simulink model "Saucer_LQG"  (R2015b)
settings: Solver=ode3  StartTime=0.0  StopTime=inf  FixedStep=0.05  RelTol=1e-3
undefined symbols (not defined in the file or in its folder): A, B, C, K_lqr, Kd, Kp, L_obs, MAPP1, MAPP2, MAPP3, pinvTr, ref, Th1, Th2, Th3
libraries: robotlib x11, realtime_pacer_lib x1
settings Model: Creator=saucer  LastModifiedBy=saucer
settings OptimizationCC: OptimizeModelRefInitCode=on  LifeSpan=Inf  MaxStackSize=64
settings HardwareCC: ProdBitPerPointer=32  ProdLargestAtomicFloat=None  ProdIntDivRoundTo=Undefined  ProdEndianess=Unspecified  ProdWordSize=32  ProdHWDeviceType=Generic->Unspecified (assume 32-bit Generic)
settings RTWCC: SystemTargetFile=ert.tlc  TemplateMakefile=ert_default_tmf  Description=Embedded Coder  Toolchain=Catkin  TargetLang=C++
settings CodeAppCC: IgnoreCustomStorageClasses=off

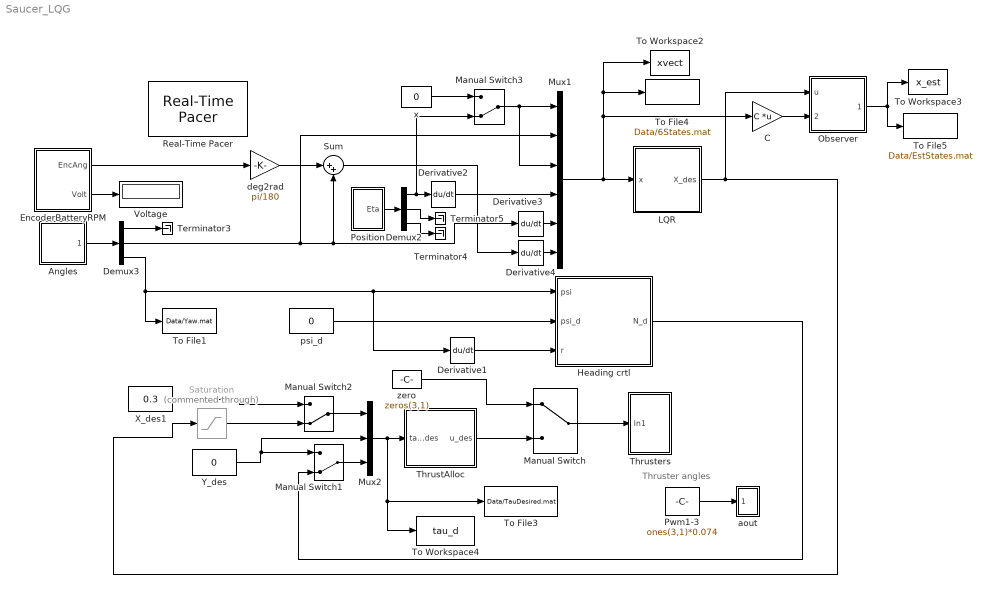
== system Saucer_LQG ==
  note: Thruster angles
  Angles : Subsystem
  C : Gain  Gain=C  Multiplication=Matrix(K*u)
  Demux2 : Demux  Outputs=3
  Demux3 : Demux  Outputs=3
  Derivative{1..4} (4 alike) : Derivative
  EncoderBatteryRPM : Subsystem
  Heading crtl : Subsystem
  LQR : Subsystem
  Manual Switch : ManualSwitch
  Manual Switch1 : ManualSwitch  CurrentSetting=0
  Manual Switch2 : ManualSwitch  CurrentSetting=0
  Manual Switch3 : ManualSwitch  CurrentSetting=0
  Mux1 : Mux  Inputs=6
  Mux2 : Mux  Inputs=3
  Observer : Subsystem
  Position : Subsystem
  Pwm1-3 : Constant  Value=ones(3,1)*0.074
  Real-Time Pacer : realtime_pacer_lib/Real-Time Pacer  simTimePerRealTime=1
  Saturation : Saturate  Commented=through  UpperLimit=3.7  LowerLimit=-3.7
  Sum : Sum  Inputs=|++
  Terminator3 : Terminator
  Terminator4 : Terminator
  Terminator5 : Terminator
  ThrustAlloc : Subsystem
  Thrusters : Subsystem
  To File1 : ToFile  Filename=Data/Yaw.mat  MatrixName=psi  SaveFormat=Timeseries
  To File3 : ToFile  Filename=Data/TauDesired.mat  MatrixName=tau_d  SaveFormat=Timeseries
  To File4 : ToFile  Filename=Data/6States.mat  MatrixName=xvect  SaveFormat=Timeseries
  To File5 : ToFile  Filename=Data/EstStates.mat  MatrixName=x_est  SaveFormat=Timeseries
  To Workspace2 : ToWorkspace  VariableName=xvect  SaveFormat=Timeseries  SampleTime=-1
  To Workspace3 : ToWorkspace  VariableName=x_est  SaveFormat=Timeseries  SampleTime=-1
  To Workspace4 : ToWorkspace  VariableName=tau_d  SaveFormat=Timeseries  SampleTime=-1
  Voltage : Display
  X_des1 : Constant  Value=0.3
  Y_des : Constant  Value=0
  aout : Subsystem
  deg2rad : Gain  Gain=pi/180
  psi_d : Constant  Value=0
  x : Constant  Value=0
  zero : Constant  Value=zeros(3,1)
  wires:
  Pwm1-3/1 -> aout/1(In1)
  ThrustAlloc/1(u_des) -> Manual Switch/2
  Mux2/1 -> ThrustAlloc/1(tau_des), To File3/1, To Workspace4/1
  EncoderBatteryRPM/1(EncAng) -> deg2rad/1
  psi_d/1 -> Heading crtl/2(psi_d)
  Y_des/1 -> Manual Switch1/1, Mux2/2
  zero/1 -> Manual Switch/1
  Derivative1/1 -> Heading crtl/3(r)
  Angles/1(EulerAng) -> Demux3/1
  Manual Switch2/1 -> Mux2/1
  Saturation/1 -> Manual Switch2/2
  X_des1/1 -> Manual Switch2/1
  Demux3/3 -> To File1/1, Heading crtl/1(psi), Derivative1/1
  Demux3/1 -> Terminator3/1
  deg2rad/1 -> Sum/1
  Demux3/2 -> Mux1/2, Derivative3/1, Sum/2
  Sum/1 -> Derivative4/1
  Demux2/2 -> Terminator5/1
  Position/1(Eta) -> Demux2/1
  Demux2/1 -> Manual Switch3/2, Derivative2/1
  Demux2/3 -> Terminator4/1
  Derivative2/1 -> Mux1/4
  Derivative3/1 -> Mux1/5
  Derivative4/1 -> Mux1/6
  Mux1/1 -> To Workspace2/1, To File4/1, C/1, LQR/1(x)
  LQR/1(X_des) -> Saturation/1, Observer/1(u)
  Manual Switch1/1 -> Mux2/3
  Heading crtl/1(N_d) -> Manual Switch1/2
  Observer/1(x_hat) -> To Workspace3/1, To File5/1
  C/1 -> Observer/2(y_tilde)
  Manual Switch3/1 -> Mux1/3, Mux1/1
  x/1 -> Manual Switch3/1
  EncoderBatteryRPM/2(Volt) -> Voltage/1
  Manual Switch/1 -> Thrusters/1(In1)

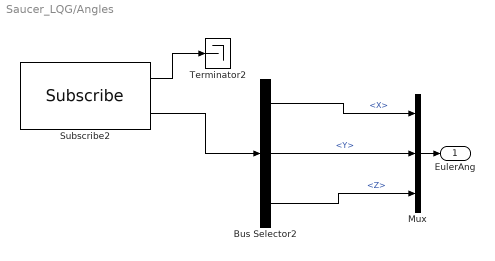
== system Saucer_LQG/Angles ==
  Bus Selector2 : BusSelector  OutputSignals=X,Y,Z
  Mux : Mux  Inputs=3
  Subscribe2 : robotlib/Subscribe  SourceLibraryInfo=This block requires Robotics System Toolbox  topicSource=Select from ROS network  topic=/EulerAng  messageType=geometry_msgs/Vector3  sampleTime=-1  messageQueueLength=1
  Terminator2 : Terminator
  EulerAng : Outport
  wires:
  Bus Selector2/3 -> Mux/3  "<Z>"
  Bus Selector2/2 -> Mux/2  "<Y>"
  Subscribe2/1 -> Terminator2/1
  Mux/1 -> EulerAng/1
  Subscribe2/2 -> Bus Selector2/1
  Bus Selector2/1 -> Mux/1  "<X>"

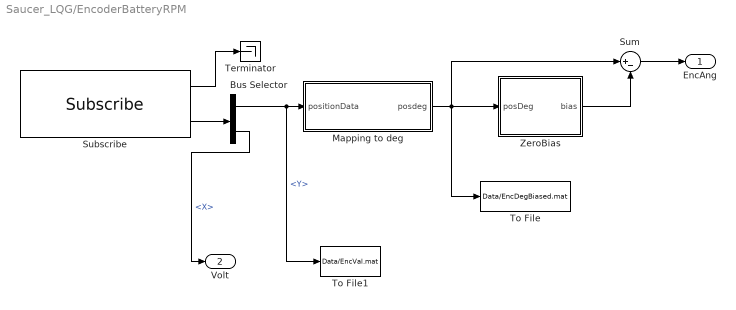
== system Saucer_LQG/EncoderBatteryRPM ==
  Bus Selector : BusSelector  OutputSignals=Linear.Y,Linear.X
  Mapping to deg : MATLAB Function  TreatAsAtomicUnit=on
  Subscribe : robotlib/Subscribe  SourceLibraryInfo=This block requires Robotics System Toolbox  topicSource=Select from ROS network  topic=/BatterEncoderThrustRPM  messageType=geometry_msgs/Twist  sampleTime=-1  messageQueueLength=1
  Sum : Sum  Inputs=|+-
  Terminator : Terminator
  To File : ToFile  Filename=Data/EncDegBiased.mat  MatrixName=EncDegBias  SaveFormat=Timeseries
  To File1 : ToFile  Filename=Data/EncVal.mat  MatrixName=EncVal  SaveFormat=Timeseries
  ZeroBias : Subsystem
  EncAng : Outport
  Volt : Outport  Port=2
  wires:
  Subscribe/1 -> Terminator/1
  ZeroBias/1(bias) -> Sum/2
  Subscribe/2 -> Bus Selector/1
  Bus Selector/1 -> To File1/1, Mapping to deg/1(positionData)  "<Y>"
  Mapping to deg/1(posdeg) -> To File/1, ZeroBias/1(posDeg), Sum/1
  Sum/1 -> EncAng/1
  Bus Selector/2 -> Volt/1  "<X>"

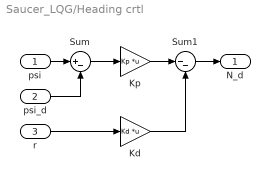
== system Saucer_LQG/Heading crtl ==
  psi : Inport
  psi_d : Inport  Port=2
  r : Inport  Port=3
  Kd : Gain  Gain=Kd  Multiplication=Matrix(K*u)
  Kp : Gain  Gain=Kp  Multiplication=Matrix(K*u)
  Sum : Sum  Inputs=|+-
  Sum1 : Sum  Inputs=|--
  N_d : Outport
  wires:
  psi/1 -> Sum/1
  psi_d/1 -> Sum/2
  Sum/1 -> Kp/1
  r/1 -> Kd/1
  Kp/1 -> Sum1/1
  Kd/1 -> Sum1/2
  Sum1/1 -> N_d/1

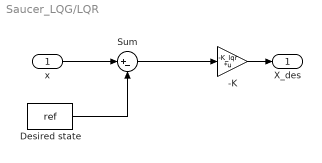
== system Saucer_LQG/LQR ==
  x : Inport
  -K : Gain  Gain=-K_lqr  Multiplication=Matrix(K*u)
  Desired state : Constant  Value=ref
  Sum : Sum  Inputs=|+-
  X_des : Outport
  wires:
  Desired state/1 -> Sum/2
  x/1 -> Sum/1
  -K/1 -> X_des/1
  Sum/1 -> -K/1

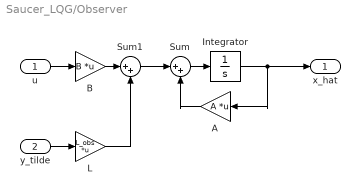
== system Saucer_LQG/Observer ==
  u : Inport
  y_tilde : Inport  Port=2
  A : Gain  Gain=A  Multiplication=Matrix(K*u)
  B : Gain  Gain=B  Multiplication=Matrix(K*u)
  Integrator : Integrator
  L : Gain  Gain=L_obs  Multiplication=Matrix(K*u)
  Sum : Sum  Inputs=|++
  Sum1 : Sum  Inputs=|++
  x_hat : Outport
  wires:
  u/1 -> B/1
  Integrator/1 -> x_hat/1, A/1
  Sum/1 -> Integrator/1
  A/1 -> Sum/2
  L/1 -> Sum1/2
  Sum1/1 -> Sum/1
  B/1 -> Sum1/1
  y_tilde/1 -> L/1

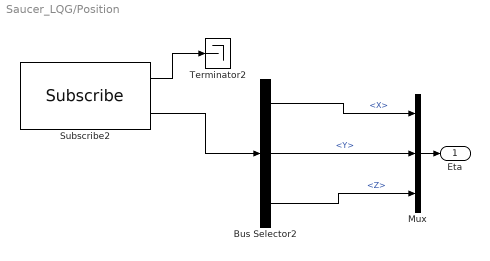
== system Saucer_LQG/Position ==
  Bus Selector2 : BusSelector  OutputSignals=X,Y,Z
  Mux : Mux  Inputs=3
  Subscribe2 : robotlib/Subscribe  SourceLibraryInfo=This block requires Robotics System Toolbox  topicSource=Select from ROS network  topic=/Eta  messageType=geometry_msgs/Vector3  sampleTime=-1  messageQueueLength=1
  Terminator2 : Terminator
  Eta : Outport
  wires:
  Bus Selector2/1 -> Mux/1  "<X>"
  Subscribe2/2 -> Bus Selector2/1
  Mux/1 -> Eta/1
  Subscribe2/1 -> Terminator2/1
  Bus Selector2/2 -> Mux/2  "<Y>"
  Bus Selector2/3 -> Mux/3  "<Z>"

== system Saucer_LQG/ThrustAlloc ==
  tau_des : Inport
  pinvTr : Gain  Gain=pinvTr  Multiplication=Matrix(K*u)
  u_des : Outport
  wires:
  pinvTr/1 -> u_des/1
  tau_des/1 -> pinvTr/1

== system Saucer_LQG/Thrusters ==
  In1 : Inport
  Data Type Conversion : DataTypeConversion  OutDataTypeStr=uint16
  EINAR2180MAP1 : Subsystem
  Idland U2PWM1 : Subsystem
  UOUT : Subsystem
  wires:
  In1/1 -> EINAR2180MAP1/1(In1), Idland U2PWM1/1(In1)
  Data Type Conversion/1 -> UOUT/1(In1)
  Idland U2PWM1/1(Out1) -> UOUT/2(U)
  EINAR2180MAP1/1(Out1) -> Data Type Conversion/1

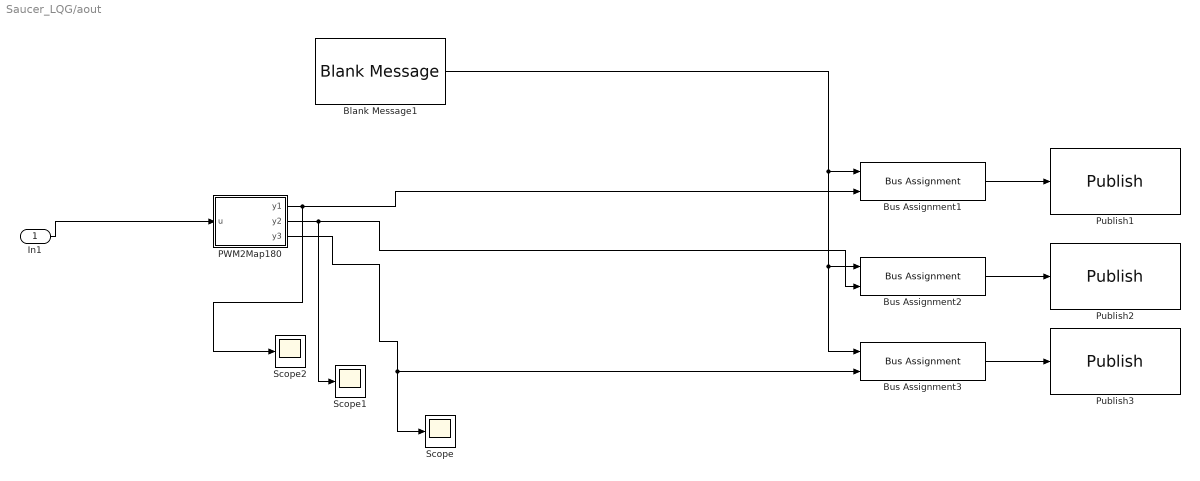
== system Saucer_LQG/aout ==
  In1 : Inport
  Blank Message1 : robotlib/Blank Message  SourceLibraryInfo=This block requires Robotics System Toolbox  messageType=std_msgs/UInt16  SampleTime=inf
  Bus Assignment1 : BusAssignment  AssignedSignals=Data
  Bus Assignment2 : BusAssignment  AssignedSignals=Data
  Bus Assignment3 : BusAssignment  AssignedSignals=Data
  "PWM2Map180 " : MATLAB Function  TreatAsAtomicUnit=on
  Publish1 : robotlib/Publish  SourceLibraryInfo=This block requires Robotics System Toolbox  topicSource=Specify your own  topic=/a1  messageType=std_msgs/UInt16  messageQueueLength=1
  Publish2 : robotlib/Publish  SourceLibraryInfo=This block requires Robotics System Toolbox  topicSource=Specify your own  topic=/a2  messageType=std_msgs/UInt16  messageQueueLength=1
  Publish3 : robotlib/Publish  SourceLibraryInfo=This block requires Robotics System Toolbox  topicSource=Specify your own  topic=/a3  messageType=std_msgs/UInt16  messageQueueLength=1
  Scope : Scope
  Scope1 : Scope
  Scope2 : Scope
  wires:
  Bus Assignment2/1 -> Publish2/1
  "PWM2Map180 "/1(y1) -> Bus Assignment1/2, Scope2/1
  "PWM2Map180 "/3(y3) -> Bus Assignment3/2, Scope/1
  In1/1 -> "PWM2Map180 "/1(u)
  Blank Message1/1 -> Bus Assignment1/1, Bus Assignment2/1, Bus Assignment3/1
  Bus Assignment1/1 -> Publish1/1
  "PWM2Map180 "/2(y2) -> Scope1/1, Bus Assignment2/2
  Bus Assignment3/1 -> Publish3/1

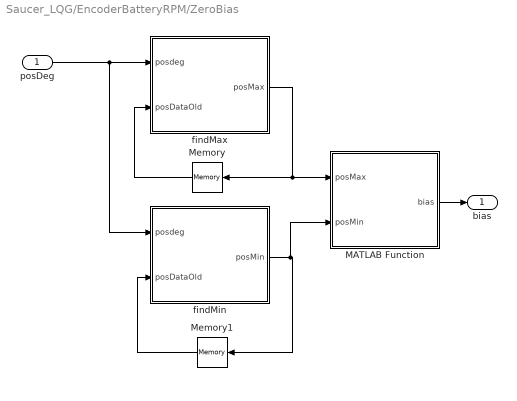
== system Saucer_LQG/EncoderBatteryRPM/ZeroBias ==
  posDeg : Inport
  MATLAB Function : MATLAB Function  TreatAsAtomicUnit=on
  Memory : Memory  X0=-360
  Memory1 : Memory  X0=360
  findMax : MATLAB Function  TreatAsAtomicUnit=on
  findMin : MATLAB Function  TreatAsAtomicUnit=on
  bias : Outport
  wires:
  findMax/1(posMax) -> Memory/1, MATLAB Function/1(posMax)
  Memory/1 -> findMax/2(posDataOld)
  Memory1/1 -> findMin/2(posDataOld)
  findMin/1(posMin) -> MATLAB Function/2(posMin), Memory1/1
  MATLAB Function/1(bias) -> bias/1
  posDeg/1 -> findMin/1(posdeg), findMax/1(posdeg)

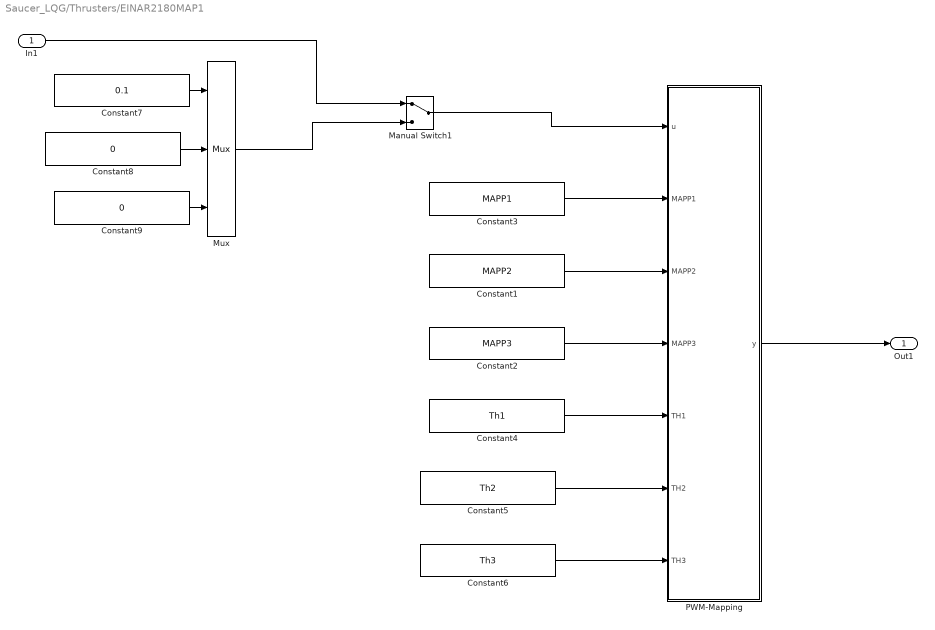
== system Saucer_LQG/Thrusters/EINAR2180MAP1 ==
  In1 : Inport
  Constant1 : Constant  Value=MAPP2
  Constant2 : Constant  Value=MAPP3
  Constant3 : Constant  Value=MAPP1
  Constant4 : Constant  Value=Th1
  Constant5 : Constant  Value=Th2
  Constant6 : Constant  Value=Th3
  Constant7 : Constant  Value=0.1
  Constant8 : Constant  Value=0
  Constant9 : Constant  Value=0
  Manual Switch1 : ManualSwitch
  Mux : Mux  Inputs=3
  PWM-Mapping : MATLAB Function  TreatAsAtomicUnit=on
  Out1 : Outport
  wires:
  Manual Switch1/1 -> PWM-Mapping/1(u)
  Constant4/1 -> PWM-Mapping/5(TH1)
  Constant6/1 -> PWM-Mapping/7(TH3)
  Constant5/1 -> PWM-Mapping/6(TH2)
  Constant3/1 -> PWM-Mapping/2(MAPP1)
  Constant1/1 -> PWM-Mapping/3(MAPP2)
  Constant2/1 -> PWM-Mapping/4(MAPP3)
  PWM-Mapping/1(y) -> Out1/1
  In1/1 -> Manual Switch1/1
  Constant7/1 -> Mux/1
  Constant8/1 -> Mux/2
  Mux/1 -> Manual Switch1/2
  Constant9/1 -> Mux/3

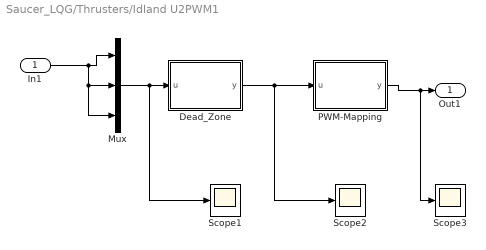
== system Saucer_LQG/Thrusters/Idland U2PWM1 ==
  In1 : Inport
  Dead_Zone : MATLAB Function  TreatAsAtomicUnit=on
  Mux : Mux  Inputs=3
  PWM-Mapping : MATLAB Function  TreatAsAtomicUnit=on
  Scope1 : Scope
  Scope2 : Scope
  Scope3 : Scope
  Out1 : Outport
  wires:
  PWM-Mapping/1(y) -> Out1/1, Scope3/1
  Mux/1 -> Dead_Zone/1(u), Scope1/1
  In1/1 -> Mux/3, Mux/2, Mux/1
  Dead_Zone/1(y) -> PWM-Mapping/1(u), Scope2/1

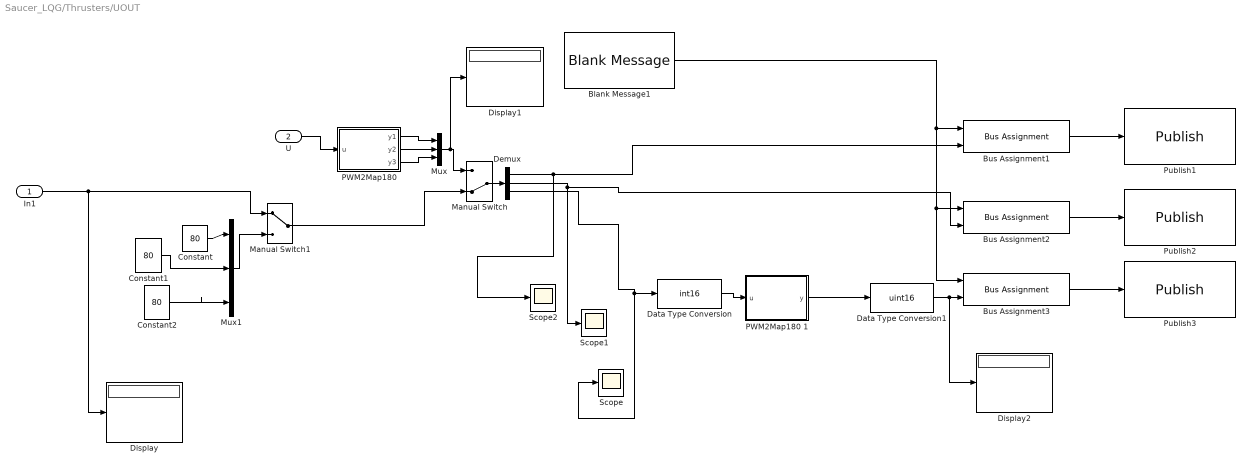
== system Saucer_LQG/Thrusters/UOUT ==
  In1 : Inport
  U : Inport  Port=2
  Blank Message1 : robotlib/Blank Message  SourceLibraryInfo=This block requires Robotics System Toolbox  messageType=std_msgs/UInt16  SampleTime=inf
  Bus Assignment1 : BusAssignment  AssignedSignals=Data
  Bus Assignment2 : BusAssignment  AssignedSignals=Data
  Bus Assignment3 : BusAssignment  AssignedSignals=Data
  Constant : Constant  Value=80  OutDataTypeStr=uint16
  Constant1 : Constant  Value=80  OutDataTypeStr=uint16
  Constant2 : Constant  Value=80  OutDataTypeStr=uint16
  Data Type Conversion : DataTypeConversion  OutDataTypeStr=int16
  Data Type Conversion1 : DataTypeConversion  OutDataTypeStr=uint16
  Demux : Demux  Outputs=3
  Display : Display
  Display1 : Display
  Display2 : Display
  Manual Switch : ManualSwitch  CurrentSetting=0
  Manual Switch1 : ManualSwitch
  Mux : Mux  Inputs=3
  Mux1 : Mux  Inputs=3
  "PWM2Map180 " : MATLAB Function  TreatAsAtomicUnit=on
  PWM2Map180 1 : MATLAB Function  TreatAsAtomicUnit=on
  Publish1 : robotlib/Publish  SourceLibraryInfo=This block requires Robotics System Toolbox  topicSource=Specify your own  topic=/Thrust1  messageType=std_msgs/UInt16  messageQueueLength=1
  Publish2 : robotlib/Publish  SourceLibraryInfo=This block requires Robotics System Toolbox  topicSource=Specify your own  topic=/Thrust2  messageType=std_msgs/UInt16  messageQueueLength=1
  Publish3 : robotlib/Publish  SourceLibraryInfo=This block requires Robotics System Toolbox  topicSource=Specify your own  topic=/Thrust3  messageType=std_msgs/UInt16  messageQueueLength=1
  Scope : Scope
  Scope1 : Scope
  Scope2 : Scope
  wires:
  Bus Assignment3/1 -> Publish3/1
  Demux/2 -> Bus Assignment2/2, Scope1/1
  Bus Assignment1/1 -> Publish1/1
  Blank Message1/1 -> Bus Assignment3/1, Bus Assignment2/1, Bus Assignment1/1
  In1/1 -> Manual Switch1/1, Display/1
  Demux/1 -> Scope2/1, Bus Assignment1/2
  Bus Assignment2/1 -> Publish2/1
  U/1 -> "PWM2Map180 "/1(u)
  "PWM2Map180 "/2(y2) -> Mux/2
  "PWM2Map180 "/3(y3) -> Mux/3
  "PWM2Map180 "/1(y1) -> Mux/1
  Mux/1 -> Display1/1, Manual Switch/1
  Manual Switch/1 -> Demux/1
  Mux1/1 -> Manual Switch1/2
  Constant/1 -> Mux1/1
  Constant1/1 -> Mux1/2
  Constant2/1 -> Mux1/3
  Manual Switch1/1 -> Manual Switch/2
  Demux/3 -> Data Type Conversion/1, Scope/1
  Data Type Conversion/1 -> PWM2Map180 1/1(u)
  Data Type Conversion1/1 -> Display2/1, Bus Assignment3/2
  PWM2Map180 1/1(y) -> Data Type Conversion1/1

== matlab function Saucer_LQG/EncoderBatteryRPM/Mapping to deg ==
  data: positionData input; posdeg output
function posdeg = val2deg(positionData)
%#codegen
puls = 2*2048; %2 channels x 2048 CPR
degpp = 360/puls; %Degrees pr. pulse.
% positionData = uint32(positionData); %Convert from double to uint32

%Convertion to signed data:
counterNBits = 12; %Bits in the encoder reading
signedThreshold = 2^(counterNBits-1); %Treshold for convertion to signed pos. values
signedData = positionData;
signedData(signedData > signedThreshold) = signedData(signedData > signedThreshold) - 2^counterNBits;

posdeg = signedData*degpp;

== matlab function Saucer_LQG/EncoderBatteryRPM/ZeroBias/findMax ==
  data: posdeg input; posMax output; posDataOld input
function posMax = findMax(posdeg,posDataOld)
posMax = posDataOld;
if posdeg > posDataOld
    posMax = posdeg;
end

== matlab function Saucer_LQG/EncoderBatteryRPM/ZeroBias/MATLAB Function ==
  data: posMax input; bias output; posMin input
function bias = normalRange(posMax,posMin)
range = posMax-posMin;
bias = posMin + range/2 +2.21; %Last + deg since zero is a bit off, i.e not equal travel to each side

== matlab function Saucer_LQG/aout/PWM2Map180  ==
  data: u input; y1 output; y2 output; y3 output
function [y1,y2,y3] = fcn(u)
%#codegen
y1=uint16((u(1)-0.027)*180/0.093);
y2=uint16((u(2)-0.027)*180/0.093);
y3=uint16((u(3)-0.027)*180/0.093);

== matlab function Saucer_LQG/EncoderBatteryRPM/ZeroBias/findMin ==
  data: posdeg input; posMin output; posDataOld input
function posMin = findMin(posdeg,posDataOld)
posMin = posDataOld;
if posdeg < posDataOld
    posMin = posdeg;
end

== matlab function Saucer_LQG/Thrusters/EINAR2180MAP1/PWM-Mapping ==
  data: u input; y output; MAPP1 input; MAPP2 input; MAPP3 input; TH1 input; TH2 input; TH3 input
function y = fcn(u,MAPP1,MAPP2,MAPP3,TH1,TH2,TH3)
y=[0 ;0;0]
u(3)=-u(3);
MAPP3=-MAPP1;
TH3=TH1

if u(1)>max(MAPP1)
    u(1)=max(MAPP1)
elseif u(1)<min(MAPP1)
u(1)=min(MAPP1);
end

if u(2)>max(MAPP2)
    u(2)=max(MAPP2)
elseif u(2)<min(MAPP2)
u(2)=min(MAPP2);
end

if u(3)>max(MAPP3)
    u(3)=max(MAPP3)
elseif u(3)<min(MAPP3)
u(3)=min(MAPP3);
end

y(1)=interp1(MAPP1,TH1,u(1))
y(2)=interp1(MAPP2,TH2,u(2))
y(3)=interp1(MAPP3,TH3,u(3))

if abs(u(1))<0.01
    y(1)=80;
end
if abs(u(2))<0.01
    y(2)=80;
end
if abs(u(3))<0.01
    y(3)=80;
end

== matlab function Saucer_LQG/Thrusters/Idland U2PWM1/Dead_Zone ==
  data: u input; y output
function y = fcn(u)
%#codegen
y=[0 ;0 ;0]
for i=1:3
if (u(i)<-0.005);
    y(i)=u(i)*0.8-0.15;
elseif (u(i)>0.005)
    y(i)=u(i)*0.8+0.15
end
end

== matlab function Saucer_LQG/Thrusters/Idland U2PWM1/PWM-Mapping ==
  data: u input; y output
function y = fcn(u)
y=(u.*0.0255)+(0.0685)
end

== matlab function Saucer_LQG/Thrusters/UOUT/PWM2Map180  ==
  data: u input; y1 output; y2 output; y3 output
function [y1,y2,y3] = fcn(u)
%#codegen
y1=uint16((u(1)-0.027)*180/0.093);
y2=uint16((u(2)-0.027)*180/0.093);
y3=uint16((u(3)-0.027)*180/0.093);

== matlab function Saucer_LQG/Thrusters/UOUT/PWM2Map180 1 ==
  data: u input; y output
function y  = fcn(u)
y=u;
if u<80
y=y+3
end
%     y=y+1;
% elseif u<80
%     y=y+3;
% end
